simulink model "FFAlgorytmRozszerzony"  (R2017a)
settings: Solver=ode113  StartTime=0.0  StopTime=10.0  RelTol=1e-6
values from neighbouring files (symbols this model uses):
  param = evalin('base','param')    [getSaveInfo.m]    (also in loadBackUp.m)
settings Model: Creator=www  LastModifiedBy=www
settings SolverCC: MaxConsecutiveMinStep=1000  AlgebraicLoopSolver=LineSearch
settings DataIOCC: SaveOutput=off  SignalLogging=off  DSMLogging=off  SaveTime=off

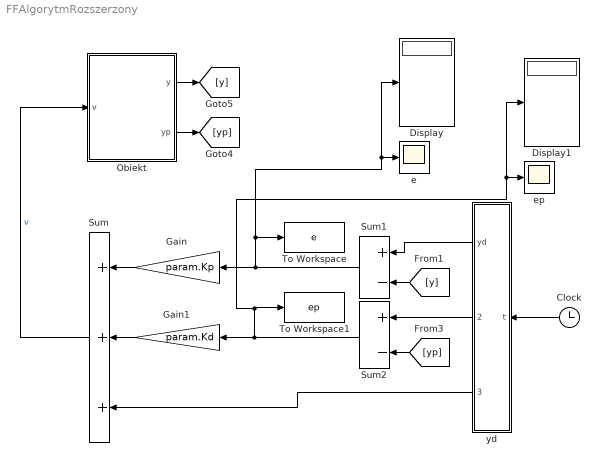
== system FFAlgorytmRozszerzony ==
  Clock : Clock
  Display : Display
  Display1 : Display
  Gain : Gain  Gain=param.Kp
  Gain1 : Gain  Gain=param.Kd
  Obiekt : Subsystem
  Sum : Sum  Inputs=+++
  Sum1 : Sum  Inputs=+-
  Sum2 : Sum  Inputs=+-
  To Workspace : ToWorkspace  VariableName=e  SaveFormat=Timeseries  SampleTime=-1
  To Workspace1 : ToWorkspace  VariableName=ep  SaveFormat=Timeseries  SampleTime=-1
  e : Scope
  ep : Scope
  yd : MATLAB Function  TreatAsAtomicUnit=on
  wires:
  Gain/1 -> Sum/1
  Obiekt/2(yp) -> [yp]
  Obiekt/1(y) -> [y]
  yd/2(ydp) -> Sum2/1
  [yp] -> Sum2/2
  [y] -> Sum1/2
  yd/1(yd) -> Sum1/1
  yd/3(ydpp) -> Sum/3
  Sum/1 -> Obiekt/1(v)  "v"
  Clock/1 -> yd/1(t)
  Sum1/1 -> Display/1, e/1, To Workspace/1, Gain/1
  Sum2/1 -> Display1/1, ep/1, To Workspace1/1, Gain1/1
  Gain1/1 -> Sum/2

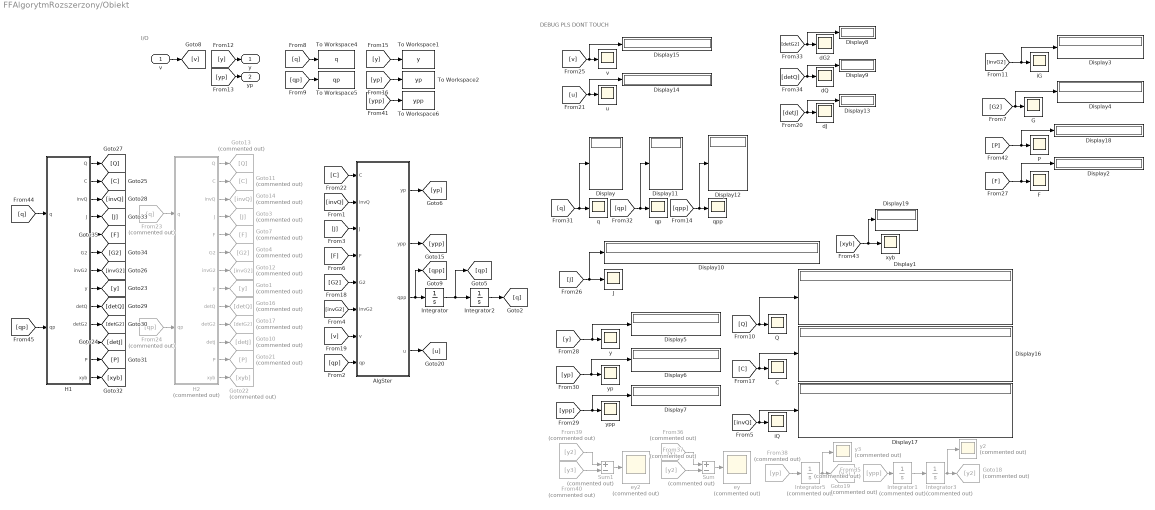
== system FFAlgorytmRozszerzony/Obiekt ==
  note: I/O
  note: DEBUG PLS DONT TOUCH
  v : Inport
  AlgSter : MATLAB Function  TreatAsAtomicUnit=on
  C : Scope
  Display{,1..19} (20 alike) : Display
  F : Scope
  From23 : From  Commented=on  GotoTag=q
  From24 : From  Commented=on  GotoTag=qp
  From35 : From  Commented=on  GotoTag=ypp
  From36 : From  Commented=on  GotoTag=y
  From37 : From  Commented=on  GotoTag=y2
  From38 : From  Commented=on  GotoTag=yp
  From39 : From  Commented=on  GotoTag=y2
  From40 : From  Commented=on  GotoTag=y3
  G : Scope
  Goto1 : Goto  Commented=on  GotoTag=y
  Goto10 : Goto  Commented=on  GotoTag=detJ
  Goto11 : Goto  Commented=on  GotoTag=C
  Goto12 : Goto  Commented=on  GotoTag=invG2
  Goto13 : Goto  Commented=on  GotoTag=Q
  Goto14 : Goto  Commented=on  GotoTag=invQ
  Goto16 : Goto  Commented=on  GotoTag=detQ
  Goto17 : Goto  Commented=on  GotoTag=detG2
  Goto18 : Goto  Commented=on  GotoTag=y2
  Goto19 : Goto  Commented=on  GotoTag=y3
  Goto21 : Goto  Commented=on  GotoTag=P
  Goto22 : Goto  Commented=on  GotoTag=xyb
  Goto3 : Goto  Commented=on  GotoTag=J
  Goto4 : Goto  Commented=on  GotoTag=G2
  Goto7 : Goto  Commented=on  GotoTag=F
  H1 : MATLAB Function  TreatAsAtomicUnit=on
  H2 : MATLAB Function  Commented=on  TreatAsAtomicUnit=on
  Integrator : Integrator  InitialCondition=param.initCond.qp0
  Integrator1 : Integrator  Commented=on  InitialCondition=param.initCond.Yp0
  Integrator2 : Integrator  InitialCondition=param.initCond.q0
  Integrator3 : Integrator  Commented=on  InitialCondition=param.initCond.Y0
  Integrator5 : Integrator  Commented=on  InitialCondition=param.initCond.Y0
  J : Scope
  P : Scope
  Q : Scope
  Sum : Sum  Commented=on  Inputs=+-
  Sum1 : Sum  Commented=on  Inputs=+-
  To Workspace1 : ToWorkspace  VariableName=y  SaveFormat=Timeseries  SampleTime=-1
  To Workspace2 : ToWorkspace  VariableName=yp  SaveFormat=Timeseries  SampleTime=-1
  To Workspace4 : ToWorkspace  VariableName=q  SaveFormat=Timeseries  SampleTime=-1
  To Workspace5 : ToWorkspace  VariableName=qp  SaveFormat=Timeseries  SampleTime=-1
  To Workspace6 : ToWorkspace  VariableName=ypp  SaveFormat=Timeseries  SampleTime=-1
  dG2 : Scope
  dJ : Scope
  dQ : Scope
  ey : Scope  Commented=on
  ey2 : Scope  Commented=on
  iG : Scope
  iQ : Scope
  q : Scope
  qp : Scope
  qpp : Scope
  "u  " : Scope
  "v  " : Scope
  xyb : Scope
  "y " : Scope
  y2 : Scope  Commented=on
  y3 : Scope  Commented=on
  "yp " : Scope
  ypp : Scope
  y : Outport
  yp : Outport  Port=2
  wires:
  v/1 -> [v]
  [G2] -> AlgSter/5(G2)
  [J] -> AlgSter/3(J)
  [v] -> AlgSter/7(v)
  [q] -> To Workspace4/1
  [yp] -> yp/1
  [yp] -> To Workspace2/1
  [y] -> To Workspace1/1
  AlgSter/2(ypp) -> [ypp]
  [y] -> y/1
  [qp] -> To Workspace5/1
  AlgSter/1(yp) -> [yp]
  [F] -> AlgSter/4(F)
  H2/6(G2) -> Goto4/1
  H2/5(F) -> Goto7/1
  From23/1 -> H2/1(q)
  From24/1 -> H2/2(qp)
  H2/2(C) -> Goto11/1
  H2/1(Q) -> Goto13/1
  H2/3(invQ) -> Goto14/1
  [C] -> AlgSter/1(C)
  [invQ] -> AlgSter/2(invQ)
  H2/8(y) -> Goto1/1
  H2/4(J) -> Goto3/1
  [qp] -> AlgSter/8(qp)
  [Q] -> Display1/1, Q/1
  [C] -> Display16/1, C/1
  [invQ] -> Display17/1, iQ/1
  [J] -> Display10/1, J/1
  [y] -> Display5/1, "y "/1
  [yp] -> Display6/1, "yp "/1
  [ypp] -> Display7/1, ypp/1
  [q] -> Display/1, q/1
  [qp] -> Display11/1, qp/1
  H2/9(detQ) -> Goto16/1
  H2/10(detG2) -> Goto17/1
  [detG2] -> Display8/1, dG2/1
  [detQ] -> Display9/1, dQ/1
  Integrator1/1 -> Integrator3/1
  From35/1 -> Integrator1/1
  Integrator3/1 -> y2/1, Goto18/1
  From36/1 -> Sum/1
  From37/1 -> Sum/2
  Sum/1 -> ey/1
  From38/1 -> Integrator5/1
  Integrator5/1 -> y3/1, Goto19/1
  From40/1 -> Sum1/2
  From39/1 -> Sum1/1
  Sum1/1 -> ey2/1
  [ypp] -> To Workspace6/1
  [F] -> Display2/1, F/1
  AlgSter/3(qpp) -> [qpp], Integrator/1
  Integrator/1 -> [qp], Integrator2/1
  Integrator2/1 -> [q]
  H2/7(invG2) -> Goto12/1
  [invG2] -> AlgSter/6(invG2)
  [invG2] -> Display3/1, iG/1
  [G2] -> Display4/1, G/1
  [qpp] -> Display12/1, qpp/1
  [detJ] -> Display13/1, dJ/1
  H2/11(detJ) -> Goto10/1
  [u] -> Display14/1, "u  "/1
  [v] -> Display15/1, "v  "/1
  AlgSter/4(u) -> [u]
  H2/12(P) -> Goto21/1
  [P] -> Display18/1, P/1
  [xyb] -> Display19/1, xyb/1
  H2/13(xyb) -> Goto22/1
  H1/13(xyb) -> [xyb]
  H1/12(P) -> [P]
  H1/11(detJ) -> [detJ]
  H1/10(detG2) -> [detG2]
  H1/3(invQ) -> [invQ]
  H1/4(J) -> [J]
  [q] -> H1/1(q)
  H1/1(Q) -> [Q]
  H1/9(detQ) -> [detQ]
  H1/8(y) -> [y]
  H1/7(invG2) -> [invG2]
  H1/5(F) -> [F]
  H1/2(C) -> [C]
  [qp] -> H1/2(qp)
  H1/6(G2) -> [G2]

== matlab function FFAlgorytmRozszerzony/Obiekt/H1 ==
  data: Q output; C output; q input; qp input; invQ output; J output; F output; G2 output; invG2 output; y output; detQ output; detG2 output; detJ output; P output; xyb output
function [Q,C,invQ,J,F,G2,invG2,y,detQ,detG2,detJ,P,xyb] = fcn(q,qp)

c0=cos(q(3));
c1=cos(q(4));
c2=cos(q(5));
s0=sin(q(3));
s1=sin(q(4));
s2=sin(q(5));
s12=sin(q(4)+q(5));
c12=cos(q(4)+q(5));
xyb=[1;1];


y=[(1/5).*(5.*q(1)+cos(q(4)+q(3))+4.*cos(q(4)+q(5)+q(3))),(1/5).*(5.*q(2)+sin( ...
  q(4)+q(3))+4.*sin(q(4)+q(5)+q(3)))];
J=[1,0,(1/5).*((-1).*sin(q(4)+q(3))+(-4).*sin(q(4)+q(5)+q(3))),(1/5).*((-1).* ...
  sin(q(4)+q(3))+(-4).*sin(q(4)+q(5)+q(3))),(-4/5).*sin(q(4)+q(5)+q(3));0,1,(1/5).*( ...
  cos(q(4)+q(3))+4.*cos(q(4)+q(5)+q(3))),(1/5).*(cos(q(4)+q(3))+4.*cos(q(4)+q(5)+q(3))),( ...
  4/5).*cos(q(4)+q(5)+q(3))];
F=[(-5).*((-365)+90.*cos(2.*q(5))).^(-1).*((qp(3)+qp(4)).^2.*cos(q(4)+q(3))+( ...
  -2).*((-3).*(qp(3)+qp(4)+qp(5)).^2.*cos(q(4)+(-1).*q(5)+q(3))+25.*(qp(3)+qp(4)+qp(5)) ...
  .^2.*cos(q(4)+q(5)+q(3))+6.*(qp(3)+qp(4)).^2.*cos(q(4)+2.*q(5)+q(3))));(-5).*((-365) ...
  +90.*cos(2.*q(5))).^(-1).*((qp(3)+qp(4)).^2.*sin(q(4)+q(3))+(-2).*((-3).*( ...
  qp(3)+qp(4)+qp(5)).^2.*sin(q(4)+(-1).*q(5)+q(3))+25.*(qp(3)+qp(4)+qp(5)).^2.*sin(q(4)+ ...
  q(5)+q(3))+6.*(qp(3)+qp(4)).^2.*sin(q(4)+2.*q(5)+q(3))))];
G2=[((-365)+90.*cos(2.*q(5))).^(-1).*(84.*sin(q(4)+q(3))+(-144).*c2.*sin( ...
  q(4)+q(5)+q(3))),6.*((-365)+90.*cos(2.*q(5))).^(-1).*((-2).*sin(q(4)+q(3))+(-3) ...
  .*sin(q(4)+(-1).*q(5)+q(3))+23.*sin(q(4)+q(5)+q(3))+12.*sin(q(4)+2.*q(5)+q(3)));(-12).* ...
  ((-365)+90.*cos(2.*q(5))).^(-1).*(cos(q(4)+q(3))+(-6).*cos(q(4)+2.*q(5)+q(3))), ...
  12.*((-365)+90.*cos(2.*q(5))).^(-1).*((7+3.*c2).*cos(q(4)+q(3))+(-1).*( ...
  13+12.*c2).*cos(q(4)+q(5)+q(3)))];
invG2=[(5/24).*((-2).*cos(q(4)+q(3))+(-3).*cos(q(4)+(-1).*q(5)+q(3))+23.*cos(q(4)+q(5)+ ...
  q(3))+12.*cos(q(4)+2.*q(5)+q(3))).*csc(q(5)),(5/24).*csc(q(5)).*((-2).*sin(q(4)+q(3)) ...
  +(-3).*sin(q(4)+(-1).*q(5)+q(3))+23.*sin(q(4)+q(5)+q(3))+12.*sin(q(4)+2.*q(5)+q(3)));( ...
  -5/12).*(cos(q(4)+q(3))+(-6).*cos(q(4)+2.*q(5)+q(3))).*csc(q(5)),(-5/12).*csc( ...
  q(5)).*(sin(q(4)+q(3))+(-6).*sin(q(4)+2.*q(5)+q(3)))];
P=[(1/5).*((-1).*(qp(3)+qp(4)).^2.*cos(q(4)+q(3))+(-4).*(qp(3)+qp(4)+qp(5)).^2.* ...
  cos(q(4)+q(5)+q(3)));(1/5).*((-1).*(qp(3)+qp(4)).^2.*sin(q(4)+q(3))+(-4).*(qp(3)+ ...
  qp(4)+qp(5)).^2.*sin(q(4)+q(5)+q(3)))];
Q=[25,0,0,0,0;0,25,0,0,0;0,0,(101/12)+2.*c2,(41/12)+2.*c2,(7/3)+ ...
  c2;0,0,(41/12)+2.*c2,(41/12)+2.*c2,(7/3)+c2;0,0,(7/3)+c2,( ...
  7/3)+c2,(7/3)];
C=[0,0,0,0,0;0,0,0,0,0;0,0,(-1).*qp(5).*s2,(-1).*qp(5).*s2,(-1).*(qp(3)+ ...
  qp(4)+qp(5)).*s2;0,0,(-1).*qp(5).*s2,(-1).*qp(5).*s2,(-1).*(qp(3)+qp(4)+ ...
  qp(5)).*s2;0,0,(qp(3)+qp(4)).*s2,(qp(3)+qp(4)).*s2,0];
invQ=[(1/25),0,0,0,0;0,(1/25),0,0,0;0,0,(1/5),(-1/5),0;0,0,(-1/5),(( ...
  -511)+36.*c2.^2).*((-365)+90.*cos(2.*q(5))).^(-1),12.*(7+3.*c2).*( ...
  (-73)+18.*cos(2.*q(5))).^(-1);0,0,0,12.*(7+3.*c2).*((-73)+18.*cos( ...
  2.*q(5))).^(-1),(-3).*(41+24.*c2).*((-73)+18.*cos(2.*q(5))).^(-1)];


detQ=det(Q);
detJ=1337;
detG2=det(G2);

== matlab function FFAlgorytmRozszerzony/Obiekt/AlgSter ==
  data: C input; invQ input; yp output; ypp output; J input; F input; G2 input; invG2 input; v input; qp input; qpp output; u output
function [yp,ypp,qpp,u] = fcn(C,invQ,J,F,G2,invG2,v,qp)

yp=J*qp;
ypp=F+G2*v;

u=invG2*(-F+v);
qpp=invQ*([0;0;0;u]-C*qp);

== matlab function FFAlgorytmRozszerzony/yd ==
  data: yd output; ydp output; ydpp output; t input
function [yd,ydp, ydpp] = fcn(t)
%id: 1atan 2poly 3sin 4cos 5const1 6const2
id=5;
id2=3;

const1=1;
const2=0;

a=-1;
b=1;

p4=3;
p3=7;
p2=16;
p1=7;
p0=1;

sina=0.02;
sinb=0.01;

cosa=-0.02;
cosb=0.02;




arctg=a*atan(b*t);
poly=p4*t^4+p3*t^3+p2*t^2+p1*t+p0;
sinn=sina*sin(sinb*t);
coss=cosa*cos(cosb*t);

polyp=4*p4*t^3+3*p3*t^2+2*p2*t+p1;
polypp=12*p4*t^2+6*p3*t+2*p2;

arctgp=(a*b)/(b^2*t^2+1);
arctgpp=-(2*a*b^3*t)/(b^2*t^2+1)^2;

sinp=sina*sinb*cos(sinb*t);
sinpp=-sina*sinb^2*sin(sinb*t);

cosp=-cosa*cosb*sin(cosb*t);
cospp=-cosa*cosb^2*cos(cosb*t);

f=[arctg,poly,sinn,coss,const1,const2];
fp=[arctgp,polyp,sinp,cosp,0,0];
fpp=[arctgpp,polypp,sinpp,cospp,0,0];

yd=[f(id);
    f(id2)];

ydp=[fp(id);
   fp(id2)];

ydpp=[fpp(id);
     fpp(id2)];

== matlab function FFAlgorytmRozszerzony/Obiekt/H2 ==
  data: Q output; C output; q input; qp input; invQ output; J output; F output; G2 output; invG2 output; y output; detQ output; detG2 output; detJ output; P output; xyb output
function [Q,C,invQ,J,F,G2,invG2,y,detQ,detG2,detJ,P,xyb] = fcn(q,qp)

c0=cos(q(3));
c1=cos(q(4));
c2=cos(q(5));
s0=sin(q(3));
s1=sin(q(4));
s2=sin(q(5));
s12=sin(q(4)+q(5));
c12=cos(q(4)+q(5));
y=[q(1)+(13/70).*cos(q(4)+q(3))+(1/7).*((-1/5).*cos(q(4)+q(3))+(-3/20).*cos( ...
  q(4)+q(5)+q(3)))+(3/10).*cos(q(4)+q(5)+q(3)),q(2)+(13/70).*sin(q(4)+q(3))+(1/7).*(( ...
  -1/5).*sin(q(4)+q(3))+(-3/20).*sin(q(4)+q(5)+q(3)))+(3/10).*sin(q(4)+q(5)+q(3))];
xb=q(1)+(-1/70).*cos(q(4)+q(3))+(1/7).*((-1/5).*cos(q(4)+q(3))+(-3/20).*cos(q(4)+ ...
  q(5)+q(3)));
yb=q(2)+(-1/70).*sin(q(4)+q(3))+(1/7).*((-1/5).*sin(q(4)+q(3))+(-3/20).*sin(q(4)+ ...
  q(5)+q(3)));
xyb=[xb;yb];


detQ=det(Q);
detJ=1337;
detG2=det(G2);
